simulink library "ChromaPowerSupply"  (R2020b)
settings: Solver=VariableStepAuto  StartTime=0.0  StopTime=10.0  RelTol=1e-3
libraries: simulink x7, fl_lib x4, nesl_utility x4, simulink_extras x1
settings Model: Creator=argol  LastModifiedBy=argol

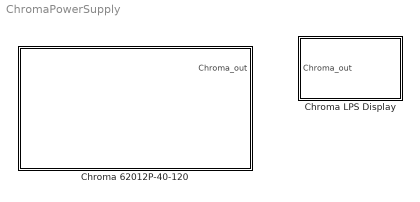
== system ChromaPowerSupply ==
  Chroma 62012P-40-120 : Subsystem  mask{set_out=1, v_out=30, i_out=20, Vmax=40, Vmin=0, Imax=120, Imin=0, Vslew=0.00001, Islew=0.00001, ttl=0, Vdcr=0, Vdcf=0, Vmax_prot=35, Imax_prot=125, Pmax_prot=1260}
      mask DialogControl DescTextVar Prompt: Chroma 62012P-40-120 Input Panel
      mask DialogControl Container16 Prompt: Output ON/OFF [0: Off, 1: ON]:
      mask DialogControl ParameterGroupVar Prompt: SETTING VOLTAGE AND CURRENT
      mask DialogControl Control23 Prompt: Set output voltage:
      mask DialogControl Control24 Prompt: Set output current:
      mask DialogControl Container26 Prompt: CONFIG
      mask DialogControl Container21 Prompt: OUTPUT SETUP
      mask DialogControl Container4 Prompt: Provide following parameters for output setup:
      mask DialogControl Control3 Prompt: Max Voltage [0~40V]:
      mask DialogControl Control4 Prompt: Min Voltage [0~40V, <Vmax]:
      mask DialogControl Control5 Prompt: Max Current [0~(+120)A]:
      mask DialogControl Control10 Prompt: Min Current [0~(+120)A, <Imax]:
      mask DialogControl Control11 Prompt: Voltage slew rate [0.000001~0.005 V/S]:
      mask DialogControl Control12 Prompt: Current slew rate [0.000001~0.001 A/S]:
      mask DialogControl Control13 Prompt: TTL Value [TBD]:
      mask DialogControl Control14 Prompt: VDC_R [TBD]:
      mask DialogControl Control15 Prompt: VDC_F [TBD]:
      mask DialogControl Container23 Prompt: PROTECTION
      mask DialogControl Container12 Prompt: Over voltage protection (OVP)
      mask DialogControl Control16 Prompt: Maximum over voltage [<=1.10*Vmax(40 V)]:
      mask DialogControl Container12_copy Prompt: Over current protection (OCP)
      mask DialogControl Control16_copy Prompt: Maximum over current [<=1.05*Imax(120 A)]:
      mask DialogControl Container12_copy_copy Prompt: Over power protection (OPP)
      mask DialogControl Control16_copy_copy Prompt: Maximum over power [<=1260 W]:
      mask Display: image('$imagefile'); % Use "Edit Image" on toolstrip to change.
  Chroma LPS Display : Subsystem
      mask DialogControl ParameterGroupVar Prompt: NHR 9200 Display block
      mask DialogControl Control2 Prompt: Look under the mask for scopes and displays

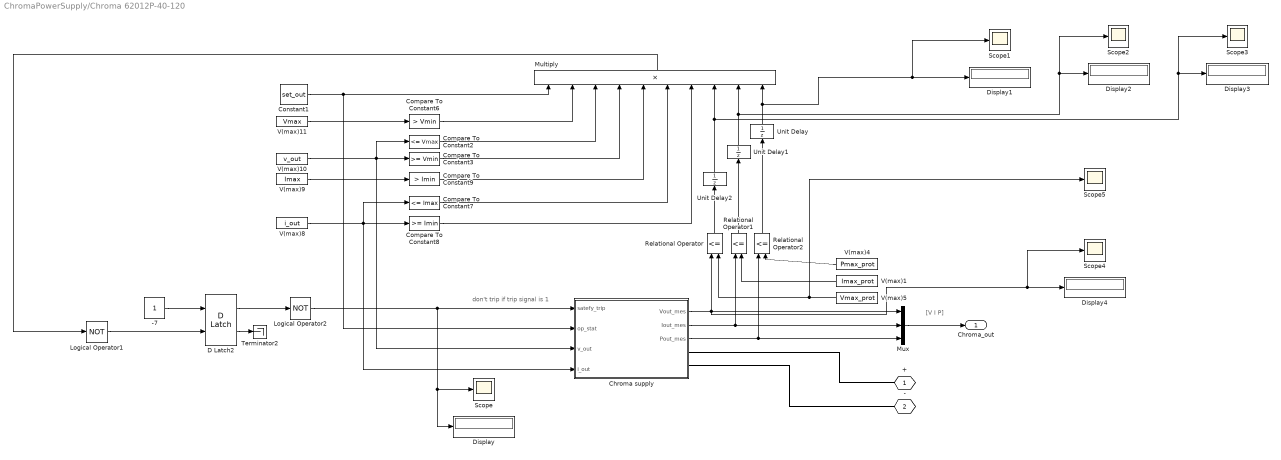
== system ChromaPowerSupply/Chroma 62012P-40-120 ==
  note: [V I P]
  note: don't trip if trip signal is 1
  -7 : Constant  OutDataTypeStr=boolean
  Chroma supply : Subsystem
  Compare To Constant2 : simulink/Logic and Bit Operations/Compare To Constant  relop=<=  const=Vmax  OutDataTypeStr=boolean
  Compare To Constant3 : simulink/Logic and Bit Operations/Compare To Constant  relop=>=  const=Vmin  OutDataTypeStr=boolean
  Compare To Constant6 : simulink/Logic and Bit Operations/Compare To Constant  relop=>  const=Vmin  OutDataTypeStr=boolean
  Compare To Constant7 : simulink/Logic and Bit Operations/Compare To Constant  relop=<=  const=Imax  OutDataTypeStr=boolean
  Compare To Constant8 : simulink/Logic and Bit Operations/Compare To Constant  relop=>=  const=Imin  OutDataTypeStr=boolean
  Compare To Constant9 : simulink/Logic and Bit Operations/Compare To Constant  relop=>  const=Imin  OutDataTypeStr=boolean
  Constant1 : Constant  Value=set_out
  D Latch2 : simulink_extras/Flip Flops/D Latch
      settings: SourceProductBaseCode=SL
  Display{,1..4} (5 alike) : Display
  Logical Operator1 : Logic  Operator=NOT  AllPortsSameDT=off  OutDataTypeStr=boolean
  Logical Operator2 : Logic  Operator=NOT  AllPortsSameDT=off  OutDataTypeStr=boolean
  Multiply : Product  Inputs=10
  Mux : Mux  Inputs=3
  Relational Operator : RelationalOperator  Operator=<=  OutDataTypeStr=boolean  RndMeth=Simplest
  Relational Operator1 : RelationalOperator  Operator=<=  OutDataTypeStr=boolean  RndMeth=Simplest
  Relational Operator2 : RelationalOperator  Operator=<=  OutDataTypeStr=boolean  RndMeth=Simplest
  Scope{,1..5} (6 alike) : Scope
  Terminator2 : Terminator
  Unit Delay : UnitDelay  InitialCondition=1  SampleTime=-1  HasFrameUpgradeWarning=on
  Unit Delay1 : UnitDelay  InitialCondition=1  SampleTime=-1  HasFrameUpgradeWarning=on
  Unit Delay2 : UnitDelay  InitialCondition=1  SampleTime=-1  HasFrameUpgradeWarning=on
  V(max)1 : Constant  Value=Imax_prot
  V(max)10 : Constant  Value=v_out
  V(max)11 : Constant  Value=Vmax
  V(max)4 : Constant  Value=Pmax_prot
  V(max)5 : Constant  Value=Vmax_prot
  V(max)8 : Constant  Value=i_out
  V(max)9 : Constant  Value=Imax
  + : PMIOPort  Side=Right
  - : PMIOPort  Port=2  Side=Right
  Chroma_out : Outport  VectorParamsAs1DForOutWhenUnconnected=off
  wires:
  V(max)11/1 -> Compare To Constant6/1
  V(max)9/1 -> Compare To Constant9/1
  Compare To Constant8/1 -> Multiply/7
  Compare To Constant7/1 -> Multiply/6
  Compare To Constant9/1 -> Multiply/5
  Compare To Constant3/1 -> Multiply/4
  Compare To Constant2/1 -> Multiply/3
  Compare To Constant6/1 -> Multiply/2
  Mux/1 -> Chroma_out/1
  V(max)8/1 -> Chroma supply/4(i_out), Compare To Constant7/1, Compare To Constant8/1
  V(max)1/1 -> Relational Operator1/2
  V(max)5/1 -> Scope5/1, Relational Operator/2
  Multiply/1 -> Logical Operator1/1
  V(max)4/1 -> Relational Operator2/2
  Constant1/1 -> Chroma supply/2("op_stat "), Multiply/1
  Chroma supply/1(Vout_mes) -> Relational Operator/1, Scope4/1, Display4/1, Mux/1
  Chroma supply/2(Iout_mes) -> Mux/2, Relational Operator1/1
  Chroma supply/3(Pout_mes) -> Mux/3, Relational Operator2/1
  Relational Operator2/1 -> Unit Delay/1
  Relational Operator1/1 -> Unit Delay1/1
  Relational Operator/1 -> Unit Delay2/1
  V(max)10/1 -> Chroma supply/3(v_out), Compare To Constant3/1, Compare To Constant2/1
  -7/1 -> D Latch2/1
  D Latch2/1 -> Logical Operator2/1
  D Latch2/2 -> Terminator2/1
  Logical Operator1/1 -> D Latch2/2
  Logical Operator2/1 -> Display/1, Scope/1, Chroma supply/1(satefy_trip)
  Unit Delay/1 -> Scope1/1, Display1/1, Multiply/10
  Unit Delay1/1 -> Scope2/1, Display2/1, Multiply/9
  Unit Delay2/1 -> Scope3/1, Display3/1, Multiply/8
  connections:
  +/RConn1 -- Chroma supply/RConn1
  Chroma supply/RConn2 -- -/RConn1

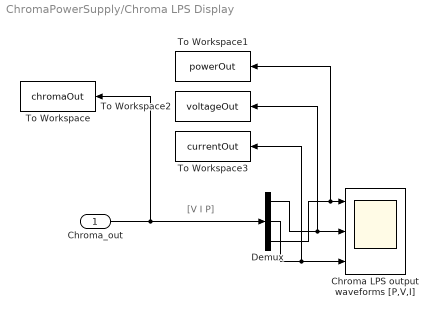
== system ChromaPowerSupply/Chroma LPS Display ==
  note: [V I P]
  Chroma_out : Inport
  Chroma LPS output waveforms [P,V,I] : Scope  NumInputPorts=3
  Demux : Demux  Outputs=3
  To Workspace : ToWorkspace  VariableName=chromaOut  SaveFormat=Timeseries  SampleTime=-1
  To Workspace1 : ToWorkspace  VariableName=powerOut  SaveFormat=Timeseries  SampleTime=-1
  To Workspace2 : ToWorkspace  VariableName=voltageOut  SaveFormat=Timeseries  SampleTime=-1
  To Workspace3 : ToWorkspace  VariableName=currentOut  SaveFormat=Timeseries  SampleTime=-1
  wires:
  Chroma_out/1 -> To Workspace/1, Demux/1
  Demux/3 -> To Workspace1/1, Chroma LPS output waveforms [P,V,I]/1
  Demux/1 -> To Workspace2/1, Chroma LPS output waveforms [P,V,I]/2
  Demux/2 -> To Workspace3/1, Chroma LPS output waveforms [P,V,I]/3

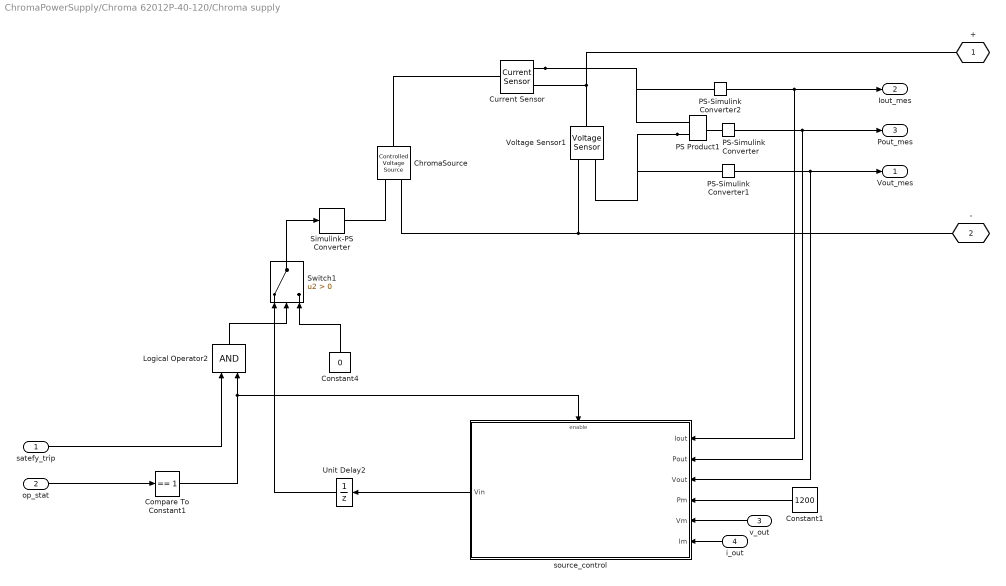
== system ChromaPowerSupply/Chroma 62012P-40-120/Chroma supply ==
  satefy_trip : Inport
  "op_stat " : Inport  Port=2
  v_out : Inport  Port=3
  i_out : Inport  Port=4
  ChromaSource : fl_lib/Electrical/Electrical Sources/Controlled Voltage Source
  Compare To Constant1 : simulink/Logic and Bit Operations/Compare To Constant  relop===  const=1  OutDataTypeStr=boolean
  Constant1 : Constant  Value=1200
  Constant4 : Constant  Value=0
  Current Sensor : fl_lib/Electrical/Electrical Sensors/Current Sensor
  Logical Operator2 : Logic  AllPortsSameDT=off  OutDataTypeStr=boolean
  PS Product1 : fl_lib/Physical Signals/Functions/PS Product
  PS-Simulink Converter : nesl_utility/PS-Simulink Converter  PhysicalDomain=network_engine_domain  SubClassName=ps_output  LeftPortType=input  RightPortType=output  PseudoPeriodic=off  Frequencies=[]  Unit=inherit  AffineConversion=off
  PS-Simulink Converter1 : nesl_utility/PS-Simulink Converter  PhysicalDomain=network_engine_domain  SubClassName=ps_output  LeftPortType=input  RightPortType=output  PseudoPeriodic=off  Frequencies=[]  Unit=inherit  AffineConversion=off
  PS-Simulink Converter2 : nesl_utility/PS-Simulink Converter  PhysicalDomain=network_engine_domain  SubClassName=ps_output  LeftPortType=input  RightPortType=output  PseudoPeriodic=off  Frequencies=[]  Unit=inherit  AffineConversion=off
  Simulink-PS Converter : nesl_utility/Simulink-PS Converter  PhysicalDomain=network_engine_domain  SubClassName=ps_input  LeftPortType=input  RightPortType=output  PseudoPeriodic=off  Frequencies=[]  NoiseDistribution=none  NoiseParameters=[]  Unit=1  AffineConversion=off  FilteringAndDerivatives=filter  SimscapeFilterOrder=1  InputFilterTimeConstant=0.001  UdotUserProvided=0
  Switch1 : Switch  Criteria=u2 > Threshold  SaturateOnIntegerOverflow=on
  Unit Delay2 : UnitDelay  InitialCondition=1  SampleTime=-1  HasFrameUpgradeWarning=on
  Voltage Sensor1 : fl_lib/Electrical/Electrical Sensors/Voltage Sensor
  source_control : Subsystem
  + : PMIOPort  Tag=PMCPort  Side=Right
  - : PMIOPort  Tag=PMCPort  Port=2  Side=Right
  Vout_mes : Outport  VectorParamsAs1DForOutWhenUnconnected=off
  Iout_mes : Outport  Port=2  VectorParamsAs1DForOutWhenUnconnected=off
  Pout_mes : Outport  Port=3  VectorParamsAs1DForOutWhenUnconnected=off
  wires:
  PS-Simulink Converter2/1 -> Iout_mes/1, source_control/1(Iout)
  PS-Simulink Converter/1 -> Pout_mes/1, source_control/2(Pout)
  PS-Simulink Converter1/1 -> Vout_mes/1, source_control/3(Vout)
  Constant4/1 -> Switch1/3
  Logical Operator2/1 -> Switch1/2
  Compare To Constant1/1 -> Logical Operator2/2, source_control/Enable
  source_control/1(Vin) -> Unit Delay2/1
  "op_stat "/1 -> Compare To Constant1/1
  Switch1/1 -> Simulink-PS Converter/1
  v_out/1 -> source_control/5(Vm)
  i_out/1 -> source_control/6(Im)
  Constant1/1 -> source_control/4(Pm)
  satefy_trip/1 -> Logical Operator2/1
  Unit Delay2/1 -> Switch1/1
  connections:
  -/RConn1 -- ChromaSource/RConn2 -- Voltage Sensor1/RConn2
  Current Sensor/RConn1 -- PS Product1/LConn1 -- PS-Simulink Converter2/LConn1
  Voltage Sensor1/LConn1 -- +/RConn1 -- Current Sensor/RConn2
  PS Product1/LConn2 -- Voltage Sensor1/RConn1 -- PS-Simulink Converter1/LConn1
  Simulink-PS Converter/RConn1 -- ChromaSource/RConn1
  ChromaSource/LConn1 -- Current Sensor/LConn1
  PS-Simulink Converter/LConn1 -- PS Product1/RConn1

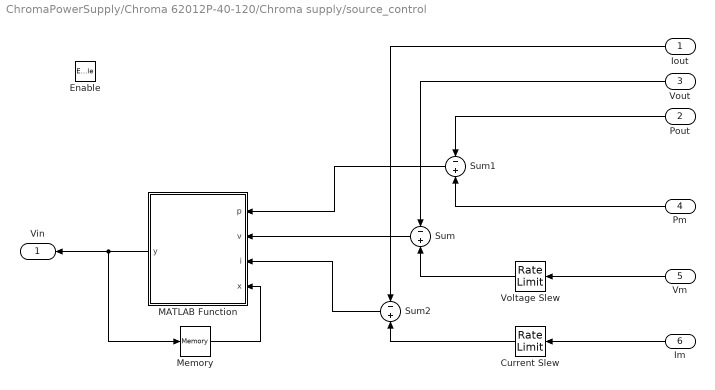
== system ChromaPowerSupply/Chroma 62012P-40-120/Chroma supply/source_control ==
  Iout : Inport
  Pout : Inport  Port=2
  Vout : Inport  Port=3
  Pm : Inport  Port=4
  Vm : Inport  Port=5
  Im : Inport  Port=6
  Enable : EnablePort
  Current Slew : RateLimiter  RisingSlewLimit=Islew  FallingSlewLimit=-Islew
  MATLAB Function : MATLAB Function  TreatAsAtomicUnit=on
  Memory : Memory
  Sum : Sum  Inputs=-+
  Sum1 : Sum  Inputs=-+
  Sum2 : Sum  Inputs=-+
  Voltage Slew : RateLimiter  RisingSlewLimit=Vslew  FallingSlewLimit=-Vslew
  Vin : Outport  VectorParamsAs1DForOutWhenUnconnected=off
  wires:
  Vout/1 -> Sum/1
  Iout/1 -> Sum2/1
  Pout/1 -> Sum1/1
  MATLAB Function/1(y) -> Memory/1, Vin/1
  Im/1 -> Current Slew/1
  Current Slew/1 -> Sum2/2
  Memory/1 -> MATLAB Function/4(x)
  Sum/1 -> MATLAB Function/2(v)
  Vm/1 -> Voltage Slew/1
  Sum1/1 -> MATLAB Function/1(p)
  Voltage Slew/1 -> Sum/2
  Sum2/1 -> MATLAB Function/3(i)
  Pm/1 -> Sum1/2

== matlab function ChromaPowerSupply/Chroma 62012P-40-120/Chroma supply/source_control/MATLAB Function ==
  data: p input; v input; y output; i input; x input
function y = fcn(p,v,i,x)
tol=1e-6;
gain=1e-4;
Ts=1e-3;
if p<=(-tol)
    y=x-(gain/Ts);
elseif i<=(-tol)
    y=x-(gain/Ts);
elseif v<=(-tol)
    y=x-(gain/Ts);
elseif v>tol;
    y=x+(gain/Ts);
else
    y=0;
end
